simulink model "vier_a"  (R2023a)
settings: Solver=VariableStepAuto  StartTime=0.0  StopTime=40  RelTol=1e-3
settings Model: Creator=alexa  LastModifiedBy=alexa

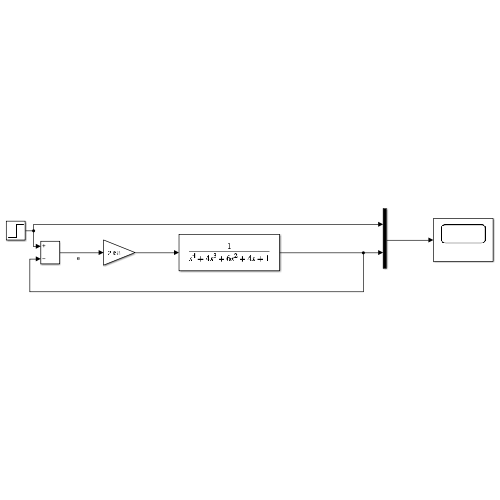
[thumbnail: Simulink's stored preview of the top-level diagram]
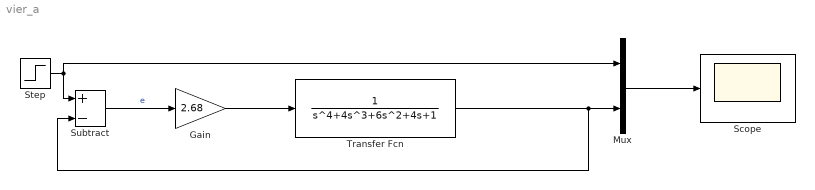
== system vier_a ==
  Gain : Gain  Gain=2.68
  Mux : Mux  Inputs=2
  Scope : Scope
  Step : Step  SampleTime=0
  Subtract : Sum  Inputs=+-
  Transfer Fcn : TransferFcn  Denominator=[1 4 6 4 1]
  wires:
  Step/1 -> Subtract/1, Mux/1
  Subtract/1 -> Gain/1  "e"
  Gain/1 -> Transfer Fcn/1
  Mux/1 -> Scope/1
  Transfer Fcn/1 -> Subtract/2, Mux/2
